simulink model "test"  (R2020b)
settings: Solver=VariableStepAuto  StartTime=0.0  StopTime=60  RelTol=1e-3
settings Model: Creator=aloks  LastModifiedBy=aloks

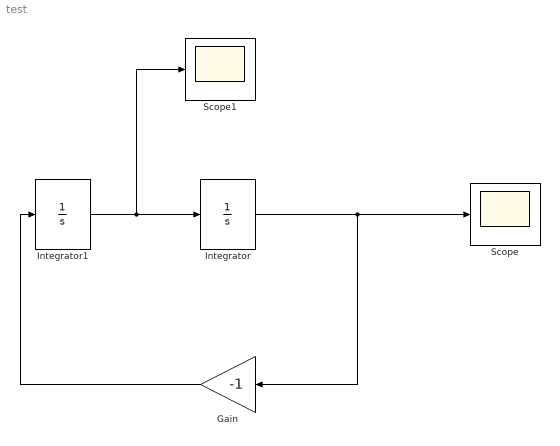
== system test ==
  Gain : Gain  Gain=-1
  Integrator : Integrator  InitialCondition=1
  Integrator1 : Integrator  InitialCondition=5
  Scope : Scope
  Scope1 : Scope
  wires:
  Integrator/1 -> Gain/1, Scope/1
  Integrator1/1 -> Scope1/1, Integrator/1
  Gain/1 -> Integrator1/1
